simulink model "translatemotion_dke"  (R2019a)
settings: Solver=VariableStepAuto  StartTime=0.0  StopTime=3000  RelTol=1e-3
values from neighbouring files (symbols this model uses):
  D = zeros(6,3)    [MPCController_test.m]
undefined symbols (not defined in the file or in its folder): attss, Continuous, protocom0303, Time
libraries: ctrlSharedLib x2, dke_attitude_ad x2, GPS_ad x1, gyros_ad x1, star_tracker_ad x1, simulink_extras x1, actuators_ad x1, dke_orbit_ad x1, cl_slector x1
settings Model: Creator=Jeong miri  LastModifiedBy=Jeong miri
settings DataIOCC: ReturnWorkspaceOutputs=off
settings DebuggingCC: ArithmeticOperatorsInVariantConditions=warning
settings SFSimCC: SimUseLocalCustomCode=off
settings RTWCC: RTWUseLocalCustomCode=off

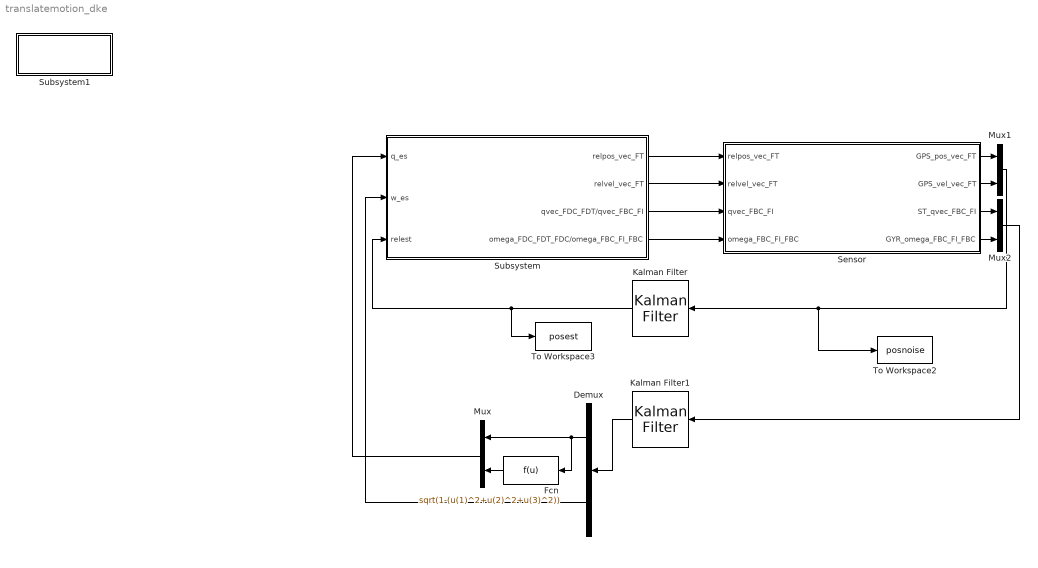
== system translatemotion_dke ==
  Demux : Demux  Outputs=2
  Fcn : Fcn  Expr=sqrt(1-(u(1)^2+u(2)^2+u(3)^2))
  Kalman Filter : ctrlSharedLib/Kalman Filter  TimeDomain=Continuous-Time  UseCurrentEstimator=on  ModelSource=Individual A, B, C, D matrices  ModelSourceVariable=sys  A=[zeros(3) eye(3); 0 0 0 0 0 0.002243; 0 -1.258e-6 0 0 0 0; 0 0 3.775e-6 -0.002243 0 0]  B=[zeros(3); 0.1*eye(3)]  C=[eye(6)]  D=[zeros(6,3)]  NumberOfStates=2  NumberOfInputs=2  NumberOfOutputs=2  InitialEstimateSource=Dialog  X0=[0 0 0 0 0 0]  P0=10*eye(3,3)  UseK=off  UseGH=off  NumberOfProcessNoiseInputs=2  G=eye(6)  TimeInvariantG=on  H=100*eye(6)  TimeInvariantH=on  Q=0.05*eye(6)  TimeInvariantQ=on  R=0.001*eye(6)  TimeInvariantR=on  N=0  TimeInvariantN=on  AddInputPort=off  AddEnablePort=off  OutputEstimatedY=off  OutputP=off  Ts=0.01
      settings: SourceProductBaseCode=CT
  Kalman Filter1 : ctrlSharedLib/Kalman Filter  TimeDomain=Continuous-Time  UseCurrentEstimator=on  ModelSource=Individual A, B, C, D matrices  ModelSourceVariable=sys  A=attss.A  B=attss.B  C=attss.C  D=attss.D  NumberOfStates=2  NumberOfInputs=2  NumberOfOutputs=2  InitialEstimateSource=Dialog  X0=[0 0 0 0 0 0]  P0=10*eye(3,3)  UseK=off  UseGH=off  NumberOfProcessNoiseInputs=2  G=eye(6)  TimeInvariantG=on  H=10*eye(6)  TimeInvariantH=on  Q=(0.25*pi/180)^2*eye(6)  TimeInvariantQ=on  R=[1e-4*eye(3) zeros(3); zeros(3) 2.5e-07*eye(3)]  TimeInvariantR=on  N=0  TimeInvariantN=on  AddInputPort=off  AddEnablePort=off  OutputEstimatedY=off  OutputP=off  Ts=0.01
      settings: SourceProductBaseCode=CT
  Mux : Mux  Inputs=2
  Mux1 : Mux  Inputs=2
  Mux2 : Mux  Inputs=2
  Sensor : Subsystem
  Subsystem : Subsystem
  Subsystem1 : Subsystem
  To Workspace2 : ToWorkspace  VariableName=posnoise  SaveFormat=Timeseries  SampleTime=-1
  To Workspace3 : ToWorkspace  VariableName=posest  SaveFormat=Timeseries  SampleTime=-1
  wires:
  Subsystem/1(relpos_vec_FT) -> Sensor/1(relpos_vec_FT)
  Subsystem/2(relvel_vec_FT) -> Sensor/2(relvel_vec_FT)
  Sensor/1(GPS_pos_vec_FT) -> Mux1/1
  Sensor/2(GPS_vel_vec_FT) -> Mux1/2
  Mux1/1 -> To Workspace2/1, Kalman Filter/1
  Kalman Filter/1 -> To Workspace3/1, Subsystem/3(relest)
  Subsystem/3(qvec_FDC_FDT/qvec_FBC_FI) -> Sensor/3(qvec_FBC_FI)
  Subsystem/4(omega_FDC_FDT_FDC/omega_FBC_FI_FBC) -> Sensor/4(omega_FBC_FI_FBC)
  Sensor/3(ST_qvec_FBC_FI) -> Mux2/1
  Sensor/4(GYR_omega_FBC_FI_FBC) -> Mux2/2
  Mux2/1 -> Kalman Filter1/1
  Kalman Filter1/1 -> Demux/1
  Demux/2 -> Subsystem/2(w_es)
  Mux/1 -> Subsystem/1(q_es)
  Demux/1 -> Fcn/1, Mux/1
  Fcn/1 -> Mux/2

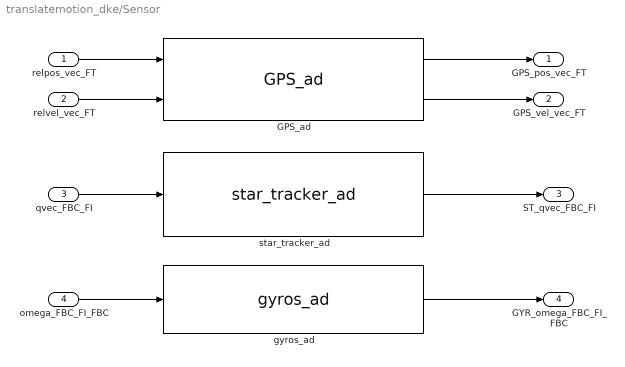
== system translatemotion_dke/Sensor ==
  relpos_vec_FT : Inport
  relvel_vec_FT : Inport  Port=2
  qvec_FBC_FI : Inport  Port=3
  omega_FBC_FI_FBC : Inport  Port=4
  GPS_ad : GPS_ad/GPS_ad  DiagCtrlNo=6  Ini_option=Specify via Dialog  InitFileName=D:\GNCDE\GPS_ad_init.m  NewFile_Action=Cancel  OldFile_Action=Cancel  InitStatus=off  GPS_ad_bias=[0,0,0,0,0,0]  GPS_ad_variance=[0.001,0.001,0.001,0.001,0.001,0.001]*0  GPS_ad_seed=[0,0,0,0,0,0]
  gyros_ad : gyros_ad/gyros_ad  DiagCtrlNo=6  Ini_option=Specify via Dialog  InitFileName=D:\GNCDE\gyros_ad_init.m  NewFile_Action=Cancel  OldFile_Action=Cancel  InitStatus=off  d_GYR1_FBC=[1 0 0]  d_GYR2_FBC=[0 1 0]  d_GYR3_FBC=[0 0 1]  GYR_ad_bias=[0 0 0]  GYR_ad_variance=[2.5e-07 2.5e-07 2.5e-07]*0  GYR_ad_seed=[0,0,0]
  star_tracker_ad : star_tracker_ad/star_tracker_ad  DiagCtrlNo=6  Ini_option=Specify via Dialog  InitFileName=D:\GNCDE\star_tracker_ad_init.m  NewFile_Action=Cancel  OldFile_Action=Cancel  InitStatus=off  ST_ad_bias=[0 0 0]  ST_ad_variance=[1e-4 1e-4 1e-4]*0  ST_ad_seed=[0,0,0]
  GPS_pos_vec_FT : Outport
  GPS_vel_vec_FT : Outport  Port=2
  ST_qvec_FBC_FI : Outport  Port=3
  GYR_omega_FBC_FI_FBC : Outport  Port=4
  wires:
  omega_FBC_FI_FBC/1 -> gyros_ad/1
  qvec_FBC_FI/1 -> star_tracker_ad/1
  gyros_ad/1 -> GYR_omega_FBC_FI_FBC/1
  GPS_ad/2 -> GPS_vel_vec_FT/1
  GPS_ad/1 -> GPS_pos_vec_FT/1
  relpos_vec_FT/1 -> GPS_ad/1
  relvel_vec_FT/1 -> GPS_ad/2
  star_tracker_ad/1 -> ST_qvec_FBC_FI/1

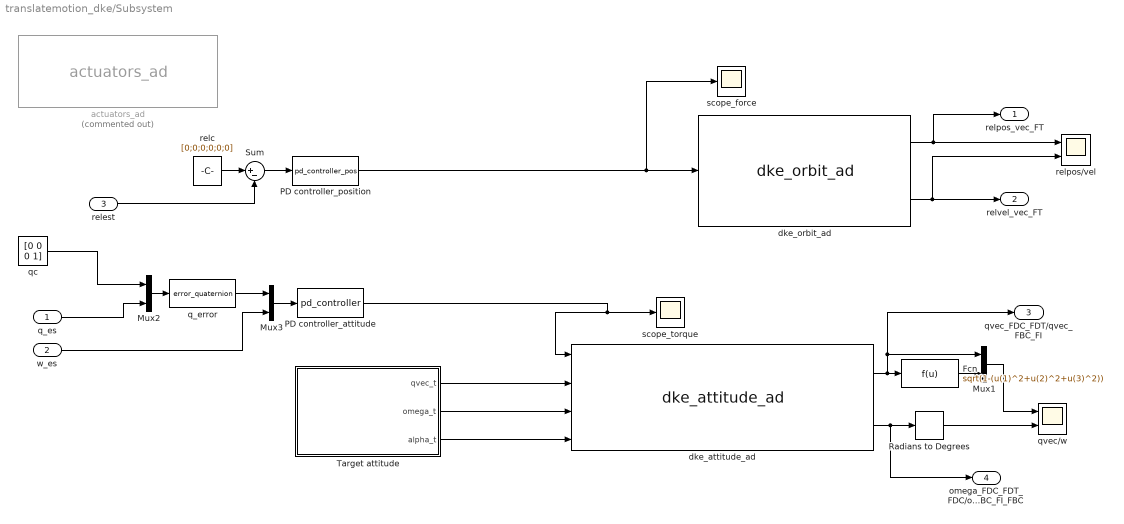
== system translatemotion_dke/Subsystem ==
  q_es : Inport
  w_es : Inport  Port=2
  relest : Inport  Port=3
  Fcn : Fcn  Expr=sqrt(1-(u(1)^2+u(2)^2+u(3)^2))
  Mux1 : Mux  Inputs=2
  Mux2 : Mux  Inputs=2
  Mux3 : Mux  Inputs=2
  PD controller_attitude : MATLABFcn  MATLABFcn=pd_controller  OutputDimensions=3
  PD controller_position : MATLABFcn  MATLABFcn=pd_controller_pos  OutputDimensions=3
  Radians to Degrees : simulink_extras/Transformations/Radians to Degrees
  Sum : Sum  Inputs=|+-
  Target attitude : Subsystem
  actuators_ad : actuators_ad/actuators_ad  Commented=on  DiagCtrlNo=6  Ini_option=Specify via Dialog  InitFileName=D:\GNCDE\working_folder\simulator\actuators_ad_init.m  NewFile_Action=Cancel  OldFile_Action=Cancel  InitStatus=off  AC_ad_bias=[0 0 0 0.00015 0.00015 0.00015]  AC_ad_variance=[0 0 0 1e-07 1e-07 1e-07]*0.1  AC_ad_seed=[0 0 0 0 0 0]
  dke_attitude_ad : dke_attitude_ad/dke_attitude_ad  DiagCtrlNo=6  Ini_option=Specify via Dialog  InitFileName=D:\GNCDE\dke_attitude_ad_init.m  NewFile_Action=Cancel  OldFile_Action=Cancel  InitStatus=off  q_FDT_FBT=[1 0 0 0]  omega_FDT_FI_FDT=[0;0;0]  C_inertia=[0.091, 0, 0;0, 0.121, 0;0, 0, 0.044]  init_qvec_FDC_FDCref="[0.0692   -0.1383    0.2075]"  init_omega_FDC_FDCref_FDC=[2 2 2]*pi/180
  dke_orbit_ad : dke_orbit_ad/dke_orbit_ad  DiagCtrlNo=6  Ini_option=Specify via Dialog  InitFileName=D:\GNCDE\dke_orbit_ad_init.m  NewFile_Action=Cancel  OldFile_Action=Cancel  InitStatus=off  C_pos_rel_FT=[0,0,0]  C_vel_rel_FT=[0,0,0]  C_ini_pos_rel_FT=[-10;0;0]  C_ini_vel_rel_FT=[0;0;0.0839]  C_mass=10  T_orbital_rate=0.0011
  q_error : MATLABFcn  MATLABFcn=error_quaternion  OutputDimensions=3
  qc : Constant  Value=[0 0 0 1]
  qvec/w : Scope  NumInputPorts=2
  relc : Constant  Value=[0;0;0;0;0;0]
  relpos/vel : Scope  NumInputPorts=2
  scope_force : Scope
  scope_torque : Scope
  relpos_vec_FT : Outport
  relvel_vec_FT : Outport  Port=2
  qvec_FDC_FDT/qvec_FBC_FI : Outport  Port=3
  omega_FDC_FDT_FDC/omega_FBC_FI_FBC : Outport  Port=4
  wires:
  dke_orbit_ad/1 -> relpos_vec_FT/1, relpos/vel/1
  relc/1 -> Sum/1
  Mux3/1 -> PD controller_attitude/1
  q_error/1 -> Mux3/1
  dke_attitude_ad/2 -> omega_FDC_FDT_FDC/omega_FBC_FI_FBC/1, Radians to Degrees/1
  dke_orbit_ad/2 -> relvel_vec_FT/1, relpos/vel/2
  Radians to Degrees/1 -> qvec/w/2
  Mux2/1 -> q_error/1
  Sum/1 -> PD controller_position/1
  Mux1/1 -> qvec/w/1
  dke_attitude_ad/1 -> Fcn/1, Mux1/1, qvec_FDC_FDT/qvec_FBC_FI/1
  w_es/1 -> Mux3/2
  q_es/1 -> Mux2/2
  relest/1 -> Sum/2
  PD controller_position/1 -> scope_force/1, dke_orbit_ad/1
  PD controller_attitude/1 -> dke_attitude_ad/1, scope_torque/1
  Fcn/1 -> Mux1/2
  Target attitude/3(alpha_t) -> dke_attitude_ad/4
  Target attitude/2(omega_t) -> dke_attitude_ad/3
  Target attitude/1(qvec_t) -> dke_attitude_ad/2
  qc/1 -> Mux2/1

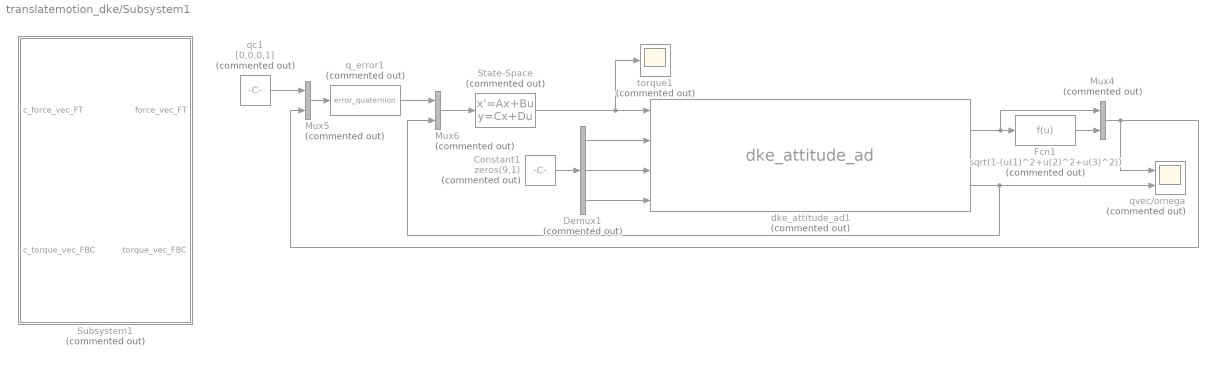
== system translatemotion_dke/Subsystem1 ==
  Constant1 : Constant  Commented=on  Value=zeros(9,1)
  Demux1 : Demux  Commented=on  Outputs=3
  Fcn1 : Fcn  Commented=on  Expr=sqrt(1-(u(1)^2+u(2)^2+u(3)^2))
  Mux4 : Mux  Commented=on  Inputs=2
  Mux5 : Mux  Commented=on  Inputs=2
  Mux6 : Mux  Commented=on  Inputs=2
  State-Space : StateSpace  Commented=on  A=zeros(6,6)  B=zeros(6,6)  C=zeros(3,6)  D=protocom0303.D  InitialCondition=0
  Subsystem1 : Subsystem  Commented=on
  dke_attitude_ad1 : dke_attitude_ad/dke_attitude_ad  Commented=on  DiagCtrlNo=6  Ini_option=Specify via Dialog  InitFileName=D:\GNCDE\dke_attitude_ad1_init.m  NewFile_Action=Cancel  OldFile_Action=Cancel  InitStatus=off  q_FDT_FBT=[1 0 0 0]  omega_FDT_FI_FDT=[0;0;0]  C_inertia=[0.091, 0, 0;0, 0.121, 0;0, 0, 0.044]  init_qvec_FDC_FDCref="[0.0692   -0.1383    0.2075]"  init_omega_FDC_FDCref_FDC=[2 2 2]*pi/180
  q_error1 : MATLABFcn  Commented=on  MATLABFcn=error_quaternion  OutputDimensions=3
  qc1 : Constant  Commented=on  Value=[0,0,0,1]
  qvec/omega : Scope  Commented=on  NumInputPorts=2
  torque1 : Scope  Commented=on
  wires:
  Mux4/1 -> qvec/omega/1, Mux5/2
  Fcn1/1 -> Mux4/2
  Constant1/1 -> Demux1/1
  Mux5/1 -> q_error1/1
  qc1/1 -> Mux5/1
  Demux1/2 -> dke_attitude_ad1/3
  Demux1/1 -> dke_attitude_ad1/2
  Demux1/3 -> dke_attitude_ad1/4
  dke_attitude_ad1/1 -> Fcn1/1, Mux4/1
  dke_attitude_ad1/2 -> qvec/omega/2, Mux6/2
  Mux6/1 -> State-Space/1
  q_error1/1 -> Mux6/1
  State-Space/1 -> torque1/1, dke_attitude_ad1/1

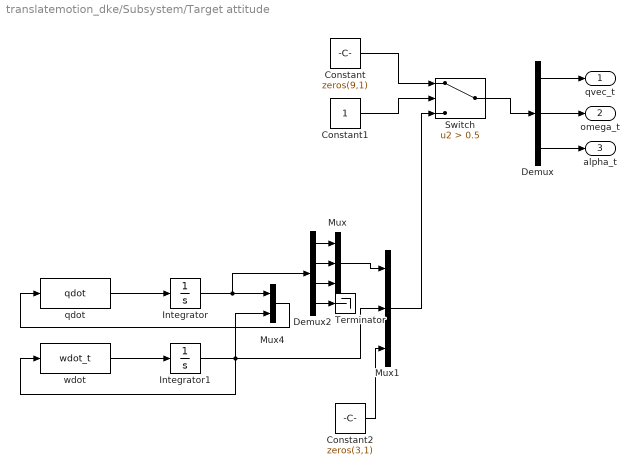
== system translatemotion_dke/Subsystem/Target attitude ==
  Constant : Constant  Value=zeros(9,1)
  Constant1 : Constant
  Constant2 : Constant  Value=zeros(3,1)
  Demux : Demux  Outputs=3
  Demux2 : Demux
  Integrator : Integrator  InitialCondition=[1 0 0 0]
  Integrator1 : Integrator  InitialCondition=[0.1 0.1 0.1]*pi/180*5
  Mux : Mux  Inputs=3
  Mux1 : Mux  Inputs=3
  Mux4 : Mux  Inputs=2
  Switch : Switch  Criteria=u2 > Threshold  Threshold=0.5
  Terminator : Terminator
  qdot : MATLABFcn  MATLABFcn=qdot
  wdot : MATLABFcn  MATLABFcn=wdot_t
  qvec_t : Outport
  omega_t : Outport  Port=2
  alpha_t : Outport  Port=3
  wires:
  Demux/3 -> alpha_t/1
  Demux/2 -> omega_t/1
  Demux/1 -> qvec_t/1
  Demux2/1 -> Mux/1
  qdot/1 -> Integrator/1
  Demux2/3 -> Mux/3
  wdot/1 -> Integrator1/1
  Demux2/4 -> Terminator/1
  Mux1/1 -> Switch/3
  Integrator1/1 -> wdot/1, Mux1/2, Mux4/2
  Mux/1 -> Mux1/1
  Mux4/1 -> qdot/1
  Demux2/2 -> Mux/2
  Integrator/1 -> Demux2/1, Mux4/1
  Switch/1 -> Demux/1
  Constant1/1 -> Switch/2
  Constant/1 -> Switch/1
  Constant2/1 -> Mux1/3

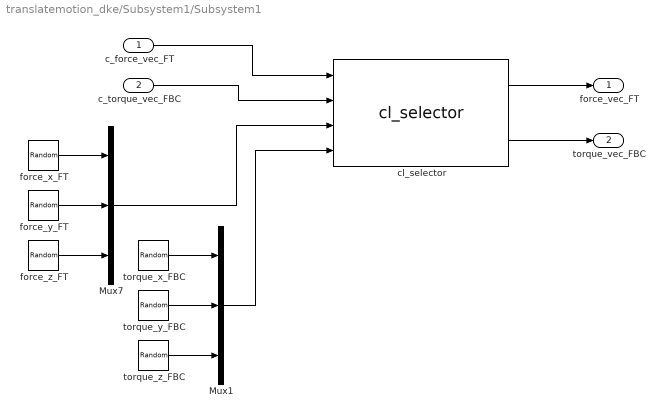
== system translatemotion_dke/Subsystem1/Subsystem1 ==
  c_force_vec_FT : Inport
  c_torque_vec_FBC : Inport  Port=2
  Mux1 : Mux  Inputs=3
  Mux7 : Mux  Inputs=3
  cl_selector : cl_slector/cl_selector  DiagCtrlNo=6  Ini_option=Specify via Dialog  InitFileName=D:\GNCDE\cl_selector_init.m  NewFile_Action=Cancel  OldFile_Action=Cancel  InitStatus=off  flag_cl_force=1  flag_cl_torque=1
  force_x_FT : RandomNumber  Variance=0.01  SampleTime=0.1
  force_y_FT : RandomNumber  Variance=0.01  Seed=1  SampleTime=0.1
  force_z_FT : RandomNumber  Variance=0.01  Seed=2  SampleTime=0.1
  torque_x_FBC : RandomNumber  Variance=0.01  SampleTime=0.1
  torque_y_FBC : RandomNumber  Variance=0.2  Seed=1  SampleTime=1
  torque_z_FBC : RandomNumber  Variance=0.2  Seed=2  SampleTime=1
  force_vec_FT : Outport
  torque_vec_FBC : Outport  Port=2
  wires:
  force_x_FT/1 -> Mux7/1
  force_z_FT/1 -> Mux7/3
  force_y_FT/1 -> Mux7/2
  Mux7/1 -> cl_selector/3
  torque_z_FBC/1 -> Mux1/3
  torque_x_FBC/1 -> Mux1/1
  Mux1/1 -> cl_selector/4
  torque_y_FBC/1 -> Mux1/2
  c_force_vec_FT/1 -> cl_selector/1
  c_torque_vec_FBC/1 -> cl_selector/2
  cl_selector/1 -> force_vec_FT/1
  cl_selector/2 -> torque_vec_FBC/1
